simulink model "Model_10_1"  (R2021a)
settings: Solver=VariableStepAuto  StartTime=0.0  StopTime=10  RelTol=1e-3
InitFcn:
  | bx=25; %25
  | bl=50; %50
  | bc=0.1; %0.08
  | 
  | ml=2; %2
  | 
  | mc=0.5;
  | M2=0.5;
  | 
  | mt=5;
  | g=9.81;
  | l_ref=0.3; %0.3
  | l_ini=1;   %1
  | l=l_ini;
  | x_ref=1; %3
  | n1=1; %5
  | n2=1;
  | 
  | L_2=0;  %chieu dai day nang ha
  | 
  | theta1_ini=0*pi/180;
  | theta2_ini=0*pi/180;  %2*pi/180
  | 
  | L_tai=0.1;
  | %ADRC' s parameter caculation
  | %b0 = (1)/(mc+mt+ml);
  | b0=(ml+mc)/(mt*mc+2*ml*mc+mt*ml+ml^2+mc^2); %Enhanced-coupling
  | %k_ESO = 100;
  | k_ESO = 100;
  | T_set  = 3; %5;
  | 
  | s_cl = -5.85/T_set;
  | Kp   = s_cl^2;
  | Kd   = -2*s_cl;
  | 
  | s_ESO = k_ESO*s_cl;
  | l1        = -3*s_ESO;
  | l2        = 3*( s_ESO)^2;
  | l3        = -(s_ESO)^3;
  | 
  | %b1 = (mt+mc)/(mc*ml +mc*mt+ml*mt);
  | b1=1/(ml+mc);
  | k_ESO1 =100; %100
  | T_set1  = 3;   %3
  | s_cl1 = -5.85/T_set1;
  | Kp1   = s_cl1^2;
  | Kd1   = -2*s_cl1;
  | 
  | s_ESO1 = k_ESO1*s_cl1;
  | l11        = -3*s_ESO1;
  | l21        = 3*( s_ESO1)^2;
  | l31        = -(s_ESO1)^3;
  | 
  | 
  | %L1=l_ini;
  | L11=0.65;
  | L2=L_tai;
  | m1=2;
  | %m2=M2;
  | m=5;
  | %Bo input shaping
  | alpha = (1/L11 + 1/L2)*(m1+M2)/m1;
  | beta = (((m1+M2)/m1)^2)*((1/L11 + 1/L2)^2) - 4*(m1+M2)/(m1*L11*L2);
  | w1 = sqrt(g*(alpha - sqrt(beta))/2);
  | w2 = sqrt(g*(alpha + sqrt(beta))/2);
  | damping_ratio = 0;
  | wd1 = w1*sqrt(1-damping_ratio^2);
  | wd2 = w2*sqrt(1-damping_ratio^2);
  | 
  | %wd1=1.998421;
  | %wd2=4.099849;
  | 
  | k = exp(damping_ratio*pi/sqrt(1-damping_ratio^2));
  | 
  | %ETM4_1
  | m_etm4_1 = 0.1;
  | I_etm4_1 = (1+m_etm4_1)*k*k/(k^2 + (1+m_etm4_1)*(k^(4/3)+k^(2/3)) + m_etm4_1);
  | A1_etm4_1 = I_etm4_1/(1+m_etm4_1);
  | A2_etm4_1 = I_etm4_1/(k^(2/3));
  | A3_etm4_1 = I_etm4_1/(k^(4/3));
  | A4_etm4_1 = m_etm4_1*I_etm4_1/((1+m_etm4_1)*(k^2));
  | t1_etm4_1 = (2*pi/3)/wd1;
  | t2_etm4_1 = (4*pi/3)/wd1;
  | t3_etm4_1 = 2*pi/wd1;
  | 
  | %ETM4_2
  | m_etm4_2 = 0.1;
  | I_etm4_2 = (1+m_etm4_2)*k*k/(k^2 + (1+m_etm4_2)*(k^(4/3)+k^(2/3)) + m_etm4_2);
  | A1_etm4_2 = I_etm4_2/(1+m_etm4_2);
  | A2_etm4_2 = I_etm4_2/(k^(2/3));
  | A3_etm4_2 = I_etm4_2/(k^(4/3));
  | A4_etm4_2 = m_etm4_2*I_etm4_2/((1+m_etm4_2)*(k^2));
  | t1_etm4_2 = (2*pi/3)/wd2;
  | t2_etm4_2 = (4*pi/3)/wd2;
  | t3_etm4_2 = 2*pi/wd2;
libraries: neural x1372, simulink x44, simulink_extras x6
(part 1 of 58)
settings Model: Creator=Dao Hieu  LastModifiedBy=Admin

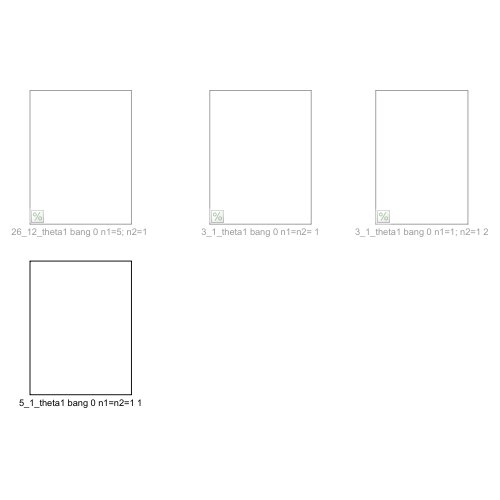
[thumbnail: Simulink's stored preview of the top-level diagram]
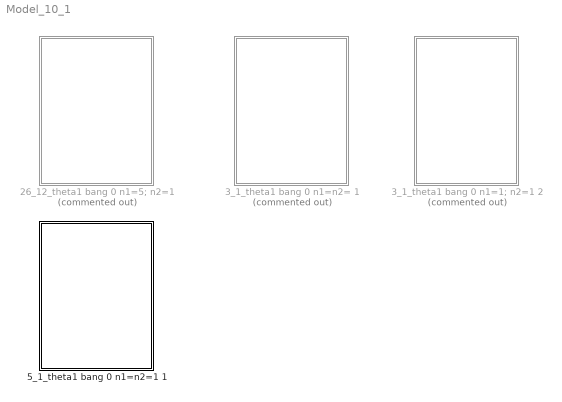
== system Model_10_1 ==
  "26_12_theta1 bang 0 n1=5; n2=1 " : Subsystem  Commented=on
  3_1_theta1 bang 0 n1=1; n2=1 2 : Subsystem  Commented=on
  3_1_theta1 bang 0 n1=n2= 1 : Subsystem  Commented=on
  5_1_theta1 bang 0 n1=n2=1 1 : Subsystem

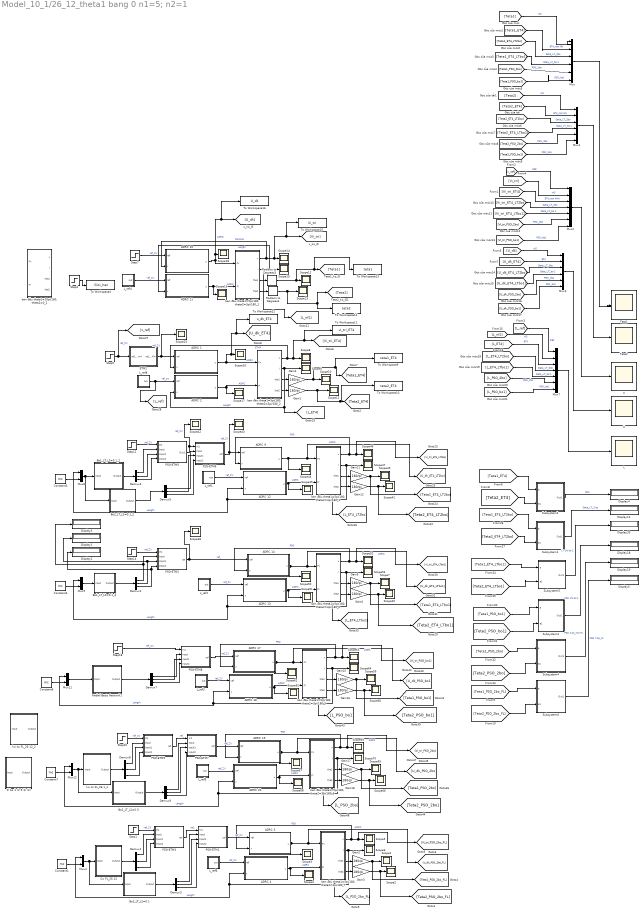
== system Model_10_1/26_12_theta1 bang 0 n1=5; n2=1  ==
  " ban đầu theta1=10pi/180, theta2=0_1" : Subsystem
  ADRC 1 : Subsystem
  ADRC 10 : Subsystem
  ADRC 11 : Subsystem
  ADRC 12 : Subsystem
  ADRC 13 : Subsystem
  ADRC 14 : Subsystem
  ADRC 17 : Subsystem
  ADRC 18 : Subsystem
  ADRC 19 : Subsystem
  ADRC 2 : Subsystem
  ADRC 20 : Subsystem
  ADRC 3 : Subsystem
  ADRC 4 : Subsystem
  ADRC 9 : Subsystem
  Bo1_LT_L2=0.1_2 : Subsystem
      mask help: Radial Basis Network
      mask Display: e = 0.06;c1 = [120 150 230]/255;c2 = ([120 150 230]+0)/383;c3 = ([120 150 230]+128)/383;patch([0 1 1 0],[0 0 1 1],c1);patch([0 1 1 1-e 1-e 0+e],[0 0 1 1-e 0+e 0+e],c2);patch([0 0 1 1-e 0+e 0+e],[0 1 1 1-e 1-e 0+e],c3);plot([0 1 1 0 0],[0 0 1 1 0]);fprintf('NNET');port_label('input',1,' Input');port_label('output',1,'Output ');
  Bo1_LT_L2=0.1_3 : Subsystem
      mask help: Radial Basis Network
      mask Display: e = 0.06;c1 = [120 150 230]/255;c2 = ([120 150 230]+0)/383;c3 = ([120 150 230]+128)/383;patch([0 1 1 0],[0 0 1 1],c1);patch([0 1 1 1-e 1-e 0+e],[0 0 1 1-e 0+e 0+e],c2);patch([0 0 1 1-e 0+e 0+e],[0 1 1 1-e 1-e 0+e],c3);plot([0 1 1 0 0],[0 0 1 1 0]);fprintf('NNET');port_label('input',1,' Input');port_label('output',1,'Output ');
  Bo2_LT_L2=0.1 : Subsystem
      mask help: Radial Basis Network
      mask Display: e = 0.06;c1 = [120 150 230]/255;c2 = ([120 150 230]+0)/383;c3 = ([120 150 230]+128)/383;patch([0 1 1 0],[0 0 1 1],c1);patch([0 1 1 1-e 1-e 0+e],[0 0 1 1-e 0+e 0+e],c2);patch([0 0 1 1-e 0+e 0+e],[0 1 1 1-e 1-e 0+e],c3);plot([0 1 1 0 0],[0 0 1 1 0]);fprintf('NNET');port_label('input',1,' Input');port_label('output',1,'Output ');
  Bo2_LT_L2=0.1_2 : Subsystem
      mask help: Radial Basis Network
      mask Display: e = 0.06;c1 = [120 150 230]/255;c2 = ([120 150 230]+0)/383;c3 = ([120 150 230]+128)/383;patch([0 1 1 0],[0 0 1 1],c1);patch([0 1 1 1-e 1-e 0+e],[0 0 1 1-e 0+e 0+e],c2);patch([0 0 1 1-e 0+e 0+e],[0 1 1 1-e 1-e 0+e],c3);plot([0 1 1 0 0],[0 0 1 1 0]);fprintf('NNET');port_label('input',1,' Input');port_label('output',1,'Output ');
  Bo2_LT_L2=0.3 : Subsystem
      mask help: Radial Basis Network
      mask Display: e = 0.06;c1 = [120 150 230]/255;c2 = ([120 150 230]+0)/383;c3 = ([120 150 230]+128)/383;patch([0 1 1 0],[0 0 1 1],c1);patch([0 1 1 1-e 1-e 0+e],[0 0 1 1-e 0+e 0+e],c2);patch([0 0 1 1-e 0+e 0+e],[0 1 1 1-e 1-e 0+e],c3);plot([0 1 1 0 0],[0 0 1 1 0]);fprintf('NNET');port_label('input',1,' Input');port_label('output',1,'Output ');
  Co FL_25.12 : Subsystem
      mask help: Radial Basis Network
      mask Display: e = 0.06;c1 = [120 150 230]/255;c2 = ([120 150 230]+0)/383;c3 = ([120 150 230]+128)/383;patch([0 1 1 0],[0 0 1 1],c1);patch([0 1 1 1-e 1-e 0+e],[0 0 1 1-e 0+e 0+e],c2);patch([0 0 1 1-e 0+e 0+e],[0 1 1 1-e 1-e 0+e],c3);plot([0 1 1 0 0],[0 0 1 1 0]);fprintf('NNET');port_label('input',1,' Input');port_label('output',1,'Output ');
  Constant{1,3..4,6..7} (5 alike) : Constant  Value=mc
  Demux{1..5,7..9} (8 alike) : Demux  Outputs=3
  Display{1..5,12,18..20} (9 alike) : Display
  ETM2 : Subsystem
  Fl bo 1 (2 5 3) (2) : Subsystem
      mask help: Radial Basis Network
      mask Display: e = 0.06;c1 = [120 150 230]/255;c2 = ([120 150 230]+0)/383;c3 = ([120 150 230]+128)/383;patch([0 1 1 0],[0 0 1 1],c1);patch([0 1 1 1-e 1-e 0+e],[0 0 1 1-e 0+e 0+e],c2);patch([0 0 1 1-e 0+e 0+e],[0 1 1 1-e 1-e 0+e],c3);plot([0 1 1 0 0],[0 0 1 1 0]);fprintf('NNET');port_label('input',1,' Input');port_label('output',1,'Output ');
  Gain{1..6,11..12,15..18} (12 alike) : Gain  Gain=180/pi
  L : Scope
  L_ref1 : Subsystem
  L_ref2 : Subsystem
  L_ref3 : Subsystem
  L_ref4 : Subsystem
  L_ref5 : Subsystem
  L_ref6 : Subsystem
  L_ref8 : Subsystem
  Mux : Mux  Inputs=6
  Mux1 : Mux  Inputs=6
  Mux{4,8..9,11..12} (5 alike) : Mux  Inputs=2
  Mux2 : Mux  Inputs=7
  Mux3 : Mux  Inputs=6
  Mux7 : Mux  Inputs=7
  PSO-ETM1 : Subsystem
  PSO-ETM2 : Subsystem
  PSO-ETM3 : Subsystem
  PSO-ETM5 : Subsystem
  PSO-ETM6 : Subsystem
  PSO-ETM7 : Subsystem
  PSO-ETM8 : Subsystem
  PSO-ETM9 : Subsystem
  Radial Basis Network1 : Subsystem
      mask help: Radial Basis Network
      mask Display: e = 0.06;c1 = [120 150 230]/255;c2 = ([120 150 230]+0)/383;c3 = ([120 150 230]+128)/383;patch([0 1 1 0],[0 0 1 1],c1);patch([0 1 1 1-e 1-e 0+e],[0 0 1 1-e 0+e 0+e],c2);patch([0 0 1 1-e 0+e 0+e],[0 1 1 1-e 1-e 0+e],c3);plot([0 1 1 0 0],[0 0 1 1 0]);fprintf('NNET');port_label('input',1,' Input');port_label('output',1,'Output ');
  Radians to Degrees3 : simulink_extras/Transformations/Radians to Degrees
  Radians to Degrees4 : simulink_extras/Transformations/Radians to Degrees
  Scope{1..20,23,40..48,50..53,59..70} (46 alike) : Scope
  Step{1,5,7,12,14,18,20} (7 alike) : Step  Time=0  After=x_ref  SampleTime=0
  Step3 : Step  Time=0  After=10  SampleTime=0
  Subsystem1 : Subsystem
  Subsystem2 : Subsystem
  Subsystem3 : Subsystem
  Subsystem4 : Subsystem
  Subsystem5 : Subsystem
  Subsystem6 : Subsystem
  Teta1 : Scope
  Teta2 : Scope
  To Workspace10 : ToWorkspace  VariableName=teta2_ET4  SaveFormat=Timeseries  SampleTime=-1
  To Workspace11 : ToWorkspace  VariableName=vi_tri_ET4  SaveFormat=Timeseries  SampleTime=-1
  To Workspace12 : ToWorkspace  VariableName=u_dk_ET4  SaveFormat=Timeseries  SampleTime=-1
  To Workspace13 : ToWorkspace  VariableName=teta1  SaveFormat=Timeseries  SampleTime=-1
  To Workspace14 : ToWorkspace  VariableName=teta2  SaveFormat=Timeseries  SampleTime=-1
  To Workspace15 : ToWorkspace  VariableName=Vi_tri  SaveFormat=Timeseries  SampleTime=-1
  To Workspace16 : ToWorkspace  VariableName=U_dk  SaveFormat=Timeseries  SampleTime=-1
  To Workspace4 : ToWorkspace  VariableName=Gioi_han  SaveFormat=Timeseries  SampleTime=-1
  To Workspace9 : ToWorkspace  VariableName=teta1_ET4  SaveFormat=Timeseries  SampleTime=-1
  U : Scope
  X : Scope
  "ban đầu theta1=5pi/180, theta2=3pi/180_1" : Subsystem
  "ban đầu theta1=5pi/180, theta2=3pi/180_2" : Subsystem
  "ban đầu theta1=5pi/180, theta2=3pi/180_3" : Subsystem
  "ban đầu theta1=5pi/180, theta2=3pi/180_4" : Subsystem
  "ban đầu theta1=5pi/180, theta2=3pi/180_5" : Subsystem
  "ban đầu theta1=5pi/180, theta2=3pi/180_6" : Subsystem
  "ban đầu theta1=5pi/180, theta2=3pi/180_7" : Subsystem
  ko co FL_25.12_2 : Subsystem
      mask help: Radial Basis Network
      mask Display: e = 0.06;c1 = [120 150 230]/255;c2 = ([120 150 230]+0)/383;c3 = ([120 150 230]+128)/383;patch([0 1 1 0],[0 0 1 1],c1);patch([0 1 1 1-e 1-e 0+e],[0 0 1 1-e 0+e 0+e],c2);patch([0 0 1 1-e 0+e 0+e],[0 1 1 1-e 1-e 0+e],c3);plot([0 1 1 0 0],[0 0 1 1 0]);fprintf('NNET');port_label('input',1,' Input');port_label('output',1,'Output ');
  ko co FL_26.1_1 : Subsystem
      mask help: Radial Basis Network
      mask Display: e = 0.06;c1 = [120 150 230]/255;c2 = ([120 150 230]+0)/383;c3 = ([120 150 230]+128)/383;patch([0 1 1 0],[0 0 1 1],c1);patch([0 1 1 1-e 1-e 0+e],[0 0 1 1-e 0+e 0+e],c2);patch([0 0 1 1-e 0+e 0+e],[0 1 1 1-e 1-e 0+e],c3);plot([0 1 1 0 0],[0 0 1 1 0]);fprintf('NNET');port_label('input',1,' Input');port_label('output',1,'Output ');
  wires:
  ADRC 2/1(u) -> "ban đầu theta1=5pi/180, theta2=3pi/180_2"/2(Fl), Scope17/1  "ADRC"
  ADRC 11/1(u) -> "ban đầu theta1=5pi/180, theta2=3pi/180_1"/2(Fl), Scope19/1  "ADRC"
  ADRC 1/1(u) -> "ban đầu theta1=5pi/180, theta2=3pi/180_2"/1(Fx), To Workspace12/1, [U_dk_ET4], Scope16/1  "ADRC"
  "ban đầu theta1=5pi/180, theta2=3pi/180_2"/1(x) -> ADRC 1/2(x), To Workspace11/1, [Vi_tri_ET4], Scope8/1  "ETM4"
  "ban đầu theta1=5pi/180, theta2=3pi/180_1"/3(the1) -> Radians to Degrees3/1
  "ban đầu theta1=5pi/180, theta2=3pi/180_2"/2(l) -> [L_ET4], ADRC 2/2(x), Scope9/1  "Length"
  "ban đầu theta1=5pi/180, theta2=3pi/180_1"/1(x) -> ADRC 10/2(x), To Workspace15/1, [Vi_tri], Scope14/1  "Position"
  L_ref4/1(out) -> ADRC 11/1(ref)  "ref_ZV"
  L_ref8/1(out) -> [L_ref], ADRC 2/1(ref)  "ref_ZV"
  "ban đầu theta1=5pi/180, theta2=3pi/180_1"/2(l) -> Scope15/1, ADRC 11/2(x), [L_nIS]  "Length"
  Step7/1 -> ADRC 10/1(ref)  "ref_ZV"
  Gain4/1 -> To Workspace9/1, [Teta1_ET4], Scope10/1
  ETM2/1(ref_ETM4) -> ADRC 1/1(ref), Scope23/1  "ref_ZV"
  Step5/1 -> [x_ref], ETM2/1(ref_ETm4)  "ref_ZV"
  ADRC 10/1(u) -> "ban đầu theta1=5pi/180, theta2=3pi/180_1"/1(Fx), To Workspace16/1, [U_dk], Scope18/1  "ADRC"
  Radians to Degrees3/1 -> To Workspace13/1, [Teta1], Scope12/1
  "ban đầu theta1=5pi/180, theta2=3pi/180_1"/4(the2) -> Radians to Degrees4/1
  "ban đầu theta1=5pi/180, theta2=3pi/180_2"/3(the1) -> Gain4/1
  Gain1/1 -> To Workspace10/1, [Teta2_ET4], Scope11/1
  "ban đầu theta1=5pi/180, theta2=3pi/180_2"/4(the2) -> Gain1/1
  Radians to Degrees4/1 -> [Teta2], To Workspace14/1, Scope13/1
  [Teta2] -> Mux1/1  "nIS"
  [U_dk] -> Mux3/1  "nIS"
  [U_dk_ET4] -> Mux3/2  "ET4"
  [Teta2_ET4] -> Mux1/2  "ET4_non NN"
  [Teta1] -> Mux/1  "nIS"
  Mux2/1 -> X/1
  Mux/1 -> Teta1/1
  Mux1/1 -> Teta2/1
  Mux3/1 -> U/1
  [Teta1_ET4] -> Mux/2  "ET4_non NN"
  Step3/1 -> To Workspace4/1
  Mux7/1 -> L/1
  "ban đầu theta1=5pi/180, theta2=3pi/180_3"/3(the1) -> Gain11/1
  "ban đầu theta1=5pi/180, theta2=3pi/180_3"/1(x) -> ADRC 9/2(x), [Vi_tri_ET4_LT2bo], Scope46/1  "PSO"
  ADRC 9/1(u) -> "ban đầu theta1=5pi/180, theta2=3pi/180_3"/1(Fx), [U_dk_ET4_LT2bo], Scope44/1  "ADRC"
  Gain12/1 -> [Teta2_ET4_LT2bo], Scope41/1
  ADRC 12/1(u) -> "ban đầu theta1=5pi/180, theta2=3pi/180_3"/2(Fl), Scope45/1  "ADRC"
  Demux4/3 -> PSO-ETM5/4(Input2)
  PSO-ETM6/1(ref) -> ADRC 9/1(ref), Scope43/1  "ref_ZV"
  "ban đầu theta1=5pi/180, theta2=3pi/180_3"/4(the2) -> Gain12/1
  Step12/1 -> PSO-ETM5/1(In1)  "ref_ZV"
  Demux5/2 -> PSO-ETM6/3(Input1)
  Demux4/2 -> PSO-ETM5/3(Input1)
  Constant3/1 -> Mux8/2
  Gain11/1 -> [Teta1_ET4_LT2bo], Scope40/1
  Demux5/3 -> PSO-ETM6/4(Input2)
  "ban đầu theta1=5pi/180, theta2=3pi/180_3"/2(l) -> Scope47/1, [L_ET4_LT2bo], ADRC 12/2(x), Mux8/1  "Length"
  Bo2_LT_L2=0.1_2/1(Output) -> Demux5/1
  PSO-ETM5/1(Out1) -> PSO-ETM6/1(In1), Scope42/1  "ref_ZV"
  Demux4/1 -> PSO-ETM5/2(Input)
  Mux8/1 -> Bo2_LT_L2=0.1_2/1(Input), Bo1_LT_L2=0.1_2/1(Input)
  Demux5/1 -> PSO-ETM6/2(Input)
  L_ref1/1(out) -> ADRC 12/1(ref)  "ref_ZV"
  Demux2/1 -> Display3/1, PSO-ETM2/2(Input)
  ADRC 13/1(u) -> "ban đầu theta1=5pi/180, theta2=3pi/180_4"/2(Fl), Scope51/1  "ADRC"
  Constant4/1 -> Mux9/2
  "ban đầu theta1=5pi/180, theta2=3pi/180_4"/2(l) -> Scope53/1, [L_ET4_LTbo1], ADRC 13/2(x), Mux9/1  "Length"
  Demux2/2 -> Display1/1, PSO-ETM2/3(Input1)
  L_ref2/1(out) -> ADRC 13/1(ref)  "ref_ZV"
  Step14/1 -> PSO-ETM2/1(In1)  "ref_ZV"
  Mux9/1 -> Bo1_LT_L2=0.1_3/1(Input)
  Demux2/3 -> Display2/1, PSO-ETM2/4(Input2)
  "ban đầu theta1=5pi/180, theta2=3pi/180_4"/4(the2) -> Gain6/1
  PSO-ETM2/1(ref) -> ADRC 14/1(ref), Scope48/1  "ref_"
  Gain5/1 -> [Teta1_ET4_LTbo1], Scope7/1
  Gain6/1 -> [Teta2_ET4_LTbo1], Scope20/1
  "ban đầu theta1=5pi/180, theta2=3pi/180_4"/3(the1) -> Gain5/1
  ADRC 14/1(u) -> Scope50/1, "ban đầu theta1=5pi/180, theta2=3pi/180_4"/1(Fx), [U_dk_ET4_LTbo1]  "ADRC"
  "ban đầu theta1=5pi/180, theta2=3pi/180_4"/1(x) -> ADRC 14/2(x), [Vi_tri_ET4_LTbo1], Scope52/1  "PSO"
  Bo1_LT_L2=0.1_3/1(Output) -> Demux2/1
  Demux7/3 -> PSO-ETM8/4(Input2)
  Demux7/1 -> PSO-ETM8/2(Input)
  Gain16/1 -> [Teta2_PSO_bo1], Scope60/1
  "ban đầu theta1=5pi/180, theta2=3pi/180_5"/4(the2) -> Gain16/1
  "ban đầu theta1=5pi/180, theta2=3pi/180_5"/3(the1) -> Gain15/1
  Constant6/1 -> Mux11/2
  Gain15/1 -> [Teta1_PSO_bo1], Scope59/1
  Demux7/2 -> PSO-ETM8/3(Input1)
  "ban đầu theta1=5pi/180, theta2=3pi/180_5"/2(l) -> Scope64/1, [L_PSO_bo1], ADRC 18/2(x), Mux11/1  "Length"
  L_ref3/1(out) -> ADRC 18/1(ref)  "ref_ZV"
  PSO-ETM8/1(ref) -> ADRC 17/1(ref)  "ref_ZV"
  Step18/1 -> PSO-ETM8/1(In1)  "ref_ZV"
  ADRC 17/1(u) -> Scope61/1, "ban đầu theta1=5pi/180, theta2=3pi/180_5"/1(Fx), [U_dk_PSO_bo1]  "ADRC"
  "ban đầu theta1=5pi/180, theta2=3pi/180_5"/1(x) -> ADRC 17/2(x), [Vi_tri_PSO_bo1], Scope63/1  "PSO"
  ADRC 18/1(u) -> "ban đầu theta1=5pi/180, theta2=3pi/180_5"/2(Fl), Scope62/1  "ADRC"
  "ban đầu theta1=5pi/180, theta2=3pi/180_6"/1(x) -> ADRC 19/2(x), [Vi_tri_PSO_2bo], Scope69/1  "PSO"
  ADRC 19/1(u) -> Scope67/1, "ban đầu theta1=5pi/180, theta2=3pi/180_6"/1(Fx), [U_dk_PSO_2bo]  "ADRC"
  "ban đầu theta1=5pi/180, theta2=3pi/180_6"/2(l) -> Scope70/1, [L_PSO_2bo], ADRC 20/2(x), Mux12/1  "Length"
  L_ref5/1(out) -> ADRC 20/1(ref)  "ref_ZV"
  Step20/1 -> PSO-ETM9/1(In1)  "ref_ZV"
  "ban đầu theta1=5pi/180, theta2=3pi/180_6"/4(the2) -> Gain18/1
  "ban đầu theta1=5pi/180, theta2=3pi/180_6"/3(the1) -> Gain17/1
  Gain17/1 -> [Teta1_PSO_2bo], Scope65/1
  Gain18/1 -> [Teta2_PSO_2bo], Scope66/1
  Constant7/1 -> Mux12/2
  ADRC 20/1(u) -> "ban đầu theta1=5pi/180, theta2=3pi/180_6"/2(Fl), Scope68/1  "ADRC"
  Bo1_LT_L2=0.1_2/1(Output) -> Demux4/1
  Radial Basis Network1/1(Output) -> Demux7/1
  Mux11/1 -> Radial Basis Network1/1(Input)
  Demux8/1 -> PSO-ETM9/2(Input)
  Demux8/2 -> PSO-ETM9/3(Input1)
  Demux8/3 -> PSO-ETM9/4(Input2)
  [Teta1_ET4_LTbo1] -> Subsystem5/1(e)
  Subsystem4/1(Out1) -> Display19/1  "PSO 2 bo_non FL"
  [Teta2_ET4_LT2bo] -> Subsystem1/2(e1)
  [Teta2_PSO_bo1] -> Subsystem3/2(e1)
  Subsystem5/1(Out1) -> Display20/1  "LT chi bo 1"
  [Teta2_ET4_LTbo1] -> Subsystem5/2(e1)
  [Teta1_PSO_2bo] -> Subsystem4/1(e)
  [Teta2_PSO_2bo] -> Subsystem4/2(e1)
  Subsystem1/1(Out1) -> Display12/1  "Data_LT_2 bo"
  Subsystem3/1(Out1) -> Display18/1  "PSO chi bo 1"
  [Teta1_PSO_bo1] -> Subsystem3/1(e)
  [Teta1_ET4_LT2bo] -> Subsystem1/1(e)
  Bo2_LT_L2=0.3/1(Output) -> Demux9/1
  Demux9/2 -> PSO-ETM7/3(Input1)
  Mux12/1 -> ko co FL_26.1_1/1(Input), Bo2_LT_L2=0.3/1(Input)
  Demux9/3 -> PSO-ETM7/4(Input2)
  Demux9/1 -> PSO-ETM7/2(Input)
  PSO-ETM9/1(ref) -> PSO-ETM7/1(In1)  "ref_"
  PSO-ETM7/1(ref) -> ADRC 19/1(ref)  "ref_ZV"
  [Teta1_ET4_LT2bo] -> Mux/3  "Data_LT_2bo"
  [Teta1_ET4_LTbo1] -> Mux/4  "Data_LT_bo 1"
  [Teta1_PSO_2bo] -> Mux/5  "PSO_2bo"
  [Teta1_PSO_bo1] -> Mux/6  "PSO_bo1"
  [Teta2_ET4_LT2bo] -> Mux1/3  "Data_LT_2bo"
  [Teta2_ET4_LTbo1] -> Mux1/4  "Data_LT_bo 1"
  [Teta2_PSO_2bo] -> Mux1/5  "PSO_2bo"
  [Teta2_PSO_bo1] -> Mux1/6  "PSO_bo1"
  [x_ref] -> Mux2/1  "REF"
  [Vi_tri] -> Mux2/2  "nIS"
  [Vi_tri_ET4] -> Mux2/3  "ET4_non ANN"
  [Vi_tri_ET4_LT2bo] -> Mux2/4  "Data_LT_2bo"
  [Vi_tri_ET4_LTbo1] -> Mux2/5  "Data_LT_bo 1"
  [Vi_tri_PSO_2bo] -> Mux2/6  "PSO_2bo"
  [Vi_tri_PSO_bo1] -> Mux2/7  "PSO_bo1"
  [U_dk_ET4_LT2bo] -> Mux3/3  "Data_LT_2bo"
  [U_dk_ET4_LTbo1] -> Mux3/4  "Data_LT_bo 1"
  [U_dk_PSO_2bo] -> Mux3/5  "PSO_2bo"
  [U_dk_PSO_bo1] -> Mux3/6  "PSO_bo1"
  [L_ref] -> Mux7/1  "REF"
  [L_nIS] -> Mux7/2  "nIS"
  [L_ET4] -> Mux7/3  "ET4"
  [L_ET4_LT2bo] -> Mux7/4  "Data_LT_2bo"
  [L_ET4_LTbo1] -> Mux7/5  "Data_LT_bo 1"
  [L_PSO_2bo] -> Mux7/6  "PSO_2bo"
  [L_PSO_bo1] -> Mux7/7  "PSO_bo1"
  [Teta1_ET4] -> Subsystem2/1(e)
  [Teta2_ET4] -> Subsystem2/2(e1)
  Subsystem2/1(Out1) -> Display4/1  "ET4"
  ko co FL_26.1_1/1(Output) -> Demux8/1
  "ban đầu theta1=5pi/180, theta2=3pi/180_7"/4(the2) -> Gain3/1
  Demux1/2 -> PSO-ETM3/3(Input1)
  PSO-ETM3/1(ref) -> PSO-ETM1/1(In1)  "ref_"
  ADRC 4/1(u) -> "ban đầu theta1=5pi/180, theta2=3pi/180_7"/2(Fl), Scope4/1  "ADRC"
  Constant1/1 -> Mux4/2
  Co FL_25.12/1(Output) -> Demux1/1
  Demux1/1 -> PSO-ETM3/2(Input)
  Demux1/3 -> PSO-ETM3/4(Input2)
  Gain3/1 -> [Teta2_PSO_2bo_FL], Scope2/1
  L_ref6/1(out) -> ADRC 4/1(ref)  "ref_ZV"
  Gain2/1 -> [Teta1_PSO_2bo_FL], Scope1/1
  "ban đầu theta1=5pi/180, theta2=3pi/180_7"/2(l) -> Scope6/1, [L_PSO_2bo_FL], ADRC 4/2(x), Mux4/1  "Length"
  "ban đầu theta1=5pi/180, theta2=3pi/180_7"/3(the1) -> Gain2/1
  "ban đầu theta1=5pi/180, theta2=3pi/180_7"/1(x) -> ADRC 3/2(x), [Vi_tri_PSO_2bo_FL], Scope5/1  "PSO"
  Step1/1 -> PSO-ETM3/1(In1)  "ref_ZV"
  Demux3/1 -> PSO-ETM1/2(Input)
  PSO-ETM1/1(ref) -> ADRC 3/1(ref)  "ref_ZV"
  ADRC 3/1(u) -> Scope3/1, "ban đầu theta1=5pi/180, theta2=3pi/180_7"/1(Fx), [U_dk_PSO_2bo_FL]  "ADRC"
  Demux3/3 -> PSO-ETM1/4(Input2)
  Mux4/1 -> Co FL_25.12/1(Input), Bo2_LT_L2=0.1/1(Input)
  Demux3/2 -> PSO-ETM1/3(Input1)
  Bo2_LT_L2=0.1/1(Output) -> Demux3/1
  [Teta2_PSO_2bo_FL] -> Subsystem6/2(e1)
  Subsystem6/1(Out1) -> Display5/1  "PSO 2 bo_FL"
  [Teta1_PSO_2bo_FL] -> Subsystem6/1(e)

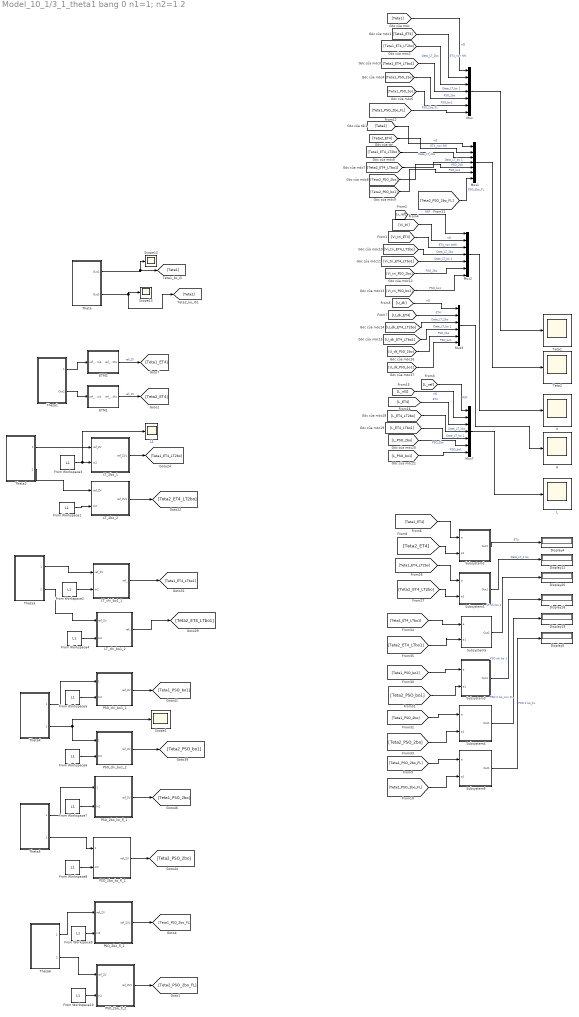
== system Model_10_1/3_1_theta1 bang 0 n1=1; n2=1 2 ==
  Display{4..5,12,18..20} (6 alike) : Display
  ETM1 : Subsystem
  ETM2 : Subsystem
  From Workspace{1..10} (10 alike) : FromWorkspace  VariableName=L1  SampleTime=5e-3
  L : Scope
  L1 : Scope
  LT_2bo_1 : Subsystem
  LT_2bo_2 : Subsystem
  LT_chi_bo1_1 : Subsystem
  LT_chi_bo1_2 : Subsystem
  Mux{,1..2,7} (4 alike) : Mux  Inputs=7
  Mux3 : Mux  Inputs=6
  PSO_2bo_fl_1 : Subsystem
  PSO_2bo_fl_2 : Subsystem
  PSO_2bo_ko_fl_1 : Subsystem
  PSO_2bo_ko_fl_2 : Subsystem
  PSO_chi_bo1_1 : Subsystem
  PSO_chi_bo1_2 : Subsystem
  Scope1 : Scope
  Scope12 : Scope
  Scope13 : Scope
  Subsystem1 : Subsystem
  Subsystem2 : Subsystem
  Subsystem3 : Subsystem
  Subsystem4 : Subsystem
  Subsystem5 : Subsystem
  Subsystem6 : Subsystem
  Teta1 : Scope
  Teta2 : Scope
  Theta : Subsystem
  Theta1 : Subsystem
  Theta2 : Subsystem
  Theta3 : Subsystem
  Theta4 : Subsystem
  Theta5 : Subsystem
  Theta6 : Subsystem
  U : Scope
  X : Scope
  wires:
  [Teta2] -> Mux1/1  "nIS"
  [U_dk] -> Mux3/1  "nIS"
  [U_dk_ET4] -> Mux3/2  "ET4"
  [Teta2_ET4] -> Mux1/2  "ET4_non NN"
  [Teta1] -> Mux/1  "nIS"
  Mux2/1 -> X/1
  Mux/1 -> Teta1/1
  Mux1/1 -> Teta2/1
  Mux3/1 -> U/1
  [Teta1_ET4] -> Mux/2  "ET4_non NN"
  Mux7/1 -> L/1
  [Teta1_ET4_LTbo1] -> Subsystem5/1(e)
  Subsystem4/1(Out1) -> Display19/1  "PSO 2 bo_non FL"
  [Teta2_ET4_LT2bo] -> Subsystem1/2(e1)
  [Teta2_PSO_bo1] -> Subsystem3/2(e1)
  Subsystem5/1(Out1) -> Display20/1  "LT chi bo 1"
  [Teta2_ET4_LTbo1] -> Subsystem5/2(e1)
  [Teta1_PSO_2bo] -> Subsystem4/1(e)
  [Teta2_PSO_2bo] -> Subsystem4/2(e1)
  Subsystem1/1(Out1) -> Display12/1  "Data_LT_2 bo"
  Subsystem3/1(Out1) -> Display18/1  "PSO chi bo 1"
  [Teta1_PSO_bo1] -> Subsystem3/1(e)
  [Teta1_ET4_LT2bo] -> Subsystem1/1(e)
  [Teta1_ET4_LT2bo] -> Mux/3  "Data_LT_2bo"
  [Teta1_ET4_LTbo1] -> Mux/4  "Data_LT_bo 1"
  [Teta1_PSO_2bo] -> Mux/5  "PSO_2bo"
  [Teta1_PSO_bo1] -> Mux/6  "PSO_bo1"
  [Teta2_ET4_LT2bo] -> Mux1/3  "Data_LT_2bo"
  [Teta2_ET4_LTbo1] -> Mux1/4  "Data_LT_bo 1"
  [Teta2_PSO_2bo] -> Mux1/5  "PSO_2bo"
  [Teta2_PSO_bo1] -> Mux1/6  "PSO_bo1"
  [x_ref] -> Mux2/1  "REF"
  [Vi_tri] -> Mux2/2  "nIS"
  [Vi_tri_ET4] -> Mux2/3  "ET4_non ANN"
  [Vi_tri_ET4_LT2bo] -> Mux2/4  "Data_LT_2bo"
  [Vi_tri_ET4_LTbo1] -> Mux2/5  "Data_LT_bo 1"
  [Vi_tri_PSO_2bo] -> Mux2/6  "PSO_2bo"
  [Vi_tri_PSO_bo1] -> Mux2/7  "PSO_bo1"
  [U_dk_ET4_LT2bo] -> Mux3/3  "Data_LT_2bo"
  [U_dk_ET4_LTbo1] -> Mux3/4  "Data_LT_bo 1"
  [U_dk_PSO_2bo] -> Mux3/5  "PSO_2bo"
  [U_dk_PSO_bo1] -> Mux3/6  "PSO_bo1"
  [L_ref] -> Mux7/1  "REF"
  [L_nIS] -> Mux7/2  "nIS"
  [L_ET4] -> Mux7/3  "ET4"
  [L_ET4_LT2bo] -> Mux7/4  "Data_LT_2bo"
  [L_ET4_LTbo1] -> Mux7/5  "Data_LT_bo 1"
  [L_PSO_2bo] -> Mux7/6  "PSO_2bo"
  [L_PSO_bo1] -> Mux7/7  "PSO_bo1"
  [Teta1_ET4] -> Subsystem2/1(e)
  [Teta2_ET4] -> Subsystem2/2(e1)
  Subsystem2/1(Out1) -> Display4/1  "ET4"
  [Teta2_PSO_2bo_FL] -> Subsystem6/2(e1)
  Subsystem6/1(Out1) -> Display5/1  "PSO 2 bo_FL"
  [Teta1_PSO_2bo_FL] -> Subsystem6/1(e)
  [Teta1_PSO_2bo_FL] -> Mux/7  "PSO_2bo_FL"
  [Teta2_PSO_2bo_FL] -> Mux1/7  "PSO_2bo_FL"
  Theta/2(Out2) -> [Teta2], Scope13/1
  Theta/1(Out1) -> Scope12/1, [Teta1]
  Theta1/1(1) -> ETM2/1(ref_ETm4)
  Theta1/2(Out2) -> ETM1/1(ref_ETm4)
  ETM2/1(ref_ETM4) -> [Teta1_ET4]  "ref_ZV"
  ETM1/1(ref_ETM4) -> [Teta2_ET4]  "ref_ZV"
  From Workspace3/1 -> L1/1, LT_2bo_1/2(In2)
  Theta2/1(1) -> LT_2bo_1/1(ref_ZV)
  Theta2/2(2) -> LT_2bo_2/1(ref_ZV)
  From Workspace1/1 -> LT_2bo_2/2(In2)
  LT_2bo_1/1(ref_ZV1) -> [Teta1_ET4_LT2bo]
  LT_2bo_2/1(ref_ZV1) -> [Teta2_ET4_LT2bo]
  Theta3/1(1) -> LT_chi_bo1_1/1(ref_ZV)
  From Workspace2/1 -> LT_chi_bo1_1/2(In2)
  LT_chi_bo1_1/1(ref_) -> [Teta1_ET4_LTbo1]
  From Workspace4/1 -> LT_chi_bo1_2/2(In2)
  Theta3/2(2) -> LT_chi_bo1_2/1(ref_ZV)
  LT_chi_bo1_2/1(ref_) -> [Teta2_ET4_LTbo1]
  From Workspace5/1 -> PSO_chi_bo1_1/2(In2)
  From Workspace6/1 -> PSO_chi_bo1_2/2(In2)
  PSO_chi_bo1_1/1(ref_ZV) -> [Teta1_PSO_bo1]
  PSO_chi_bo1_2/1(ref_ZV) -> [Teta2_PSO_bo1]
  Theta4/1(1) -> PSO_chi_bo1_1/1(1)
  Theta4/2(2) -> PSO_chi_bo1_2/1(1), Scope1/1
  From Workspace7/1 -> PSO_2bo_ko_fl_1/2(In2)
  From Workspace8/1 -> PSO_2bo_ko_fl_2/2(In2)
  Theta5/1(1) -> PSO_2bo_ko_fl_1/1(1)
  Theta5/2(2) -> PSO_2bo_ko_fl_2/1(1)
  PSO_2bo_ko_fl_1/1(ref_ZV) -> [Teta1_PSO_2bo]
  PSO_2bo_ko_fl_2/1(ref_ZV) -> [Teta2_PSO_2bo]
  From Workspace9/1 -> PSO_2bo_fl_1/2(In2)
  From Workspace10/1 -> PSO_2bo_fl_2/2(In2)
  Theta6/1(1) -> PSO_2bo_fl_1/1(ref_ZV)
  Theta6/2(2) -> PSO_2bo_fl_2/1(ref_ZV)
  PSO_2bo_fl_1/1(ref_ZV1) -> [Teta1_PSO_2bo_FL]
  PSO_2bo_fl_2/1(ref_ZV1) -> [Teta2_PSO_2bo_FL]

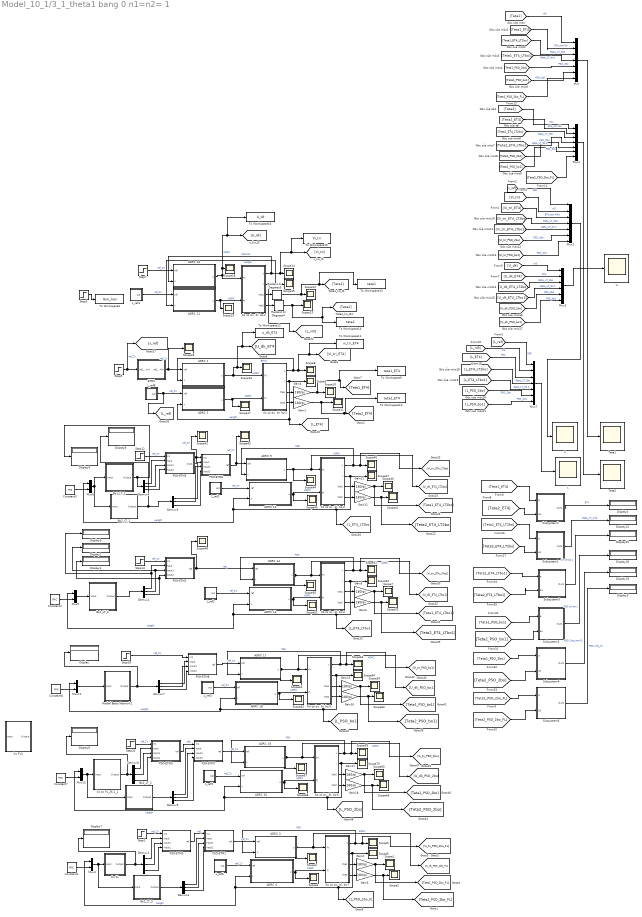
== system Model_10_1/3_1_theta1 bang 0 n1=n2= 1 ==
  ADRC 1 : Subsystem
  ADRC 10 : Subsystem
  ADRC 11 : Subsystem
  ADRC 12 : Subsystem
  ADRC 13 : Subsystem
  ADRC 14 : Subsystem
  ADRC 17 : Subsystem
  ADRC 18 : Subsystem
  ADRC 19 : Subsystem
  ADRC 2 : Subsystem
  ADRC 20 : Subsystem
  ADRC 3 : Subsystem
  ADRC 4 : Subsystem
  ADRC 9 : Subsystem
  Bo1_LT_1 : Subsystem
      mask help: Radial Basis Network
      mask Display: e = 0.06;c1 = [120 150 230]/255;c2 = ([120 150 230]+0)/383;c3 = ([120 150 230]+128)/383;patch([0 1 1 0],[0 0 1 1],c1);patch([0 1 1 1-e 1-e 0+e],[0 0 1 1-e 0+e 0+e],c2);patch([0 0 1 1-e 0+e 0+e],[0 1 1 1-e 1-e 0+e],c3);plot([0 1 1 0 0],[0 0 1 1 0]);fprintf('NNET');port_label('input',1,' Input');port_label('output',1,'Output ');
  Bo1_LT_2 : Subsystem
      mask help: Radial Basis Network
      mask Display: e = 0.06;c1 = [120 150 230]/255;c2 = ([120 150 230]+0)/383;c3 = ([120 150 230]+128)/383;patch([0 1 1 0],[0 0 1 1],c1);patch([0 1 1 1-e 1-e 0+e],[0 0 1 1-e 0+e 0+e],c2);patch([0 0 1 1-e 0+e 0+e],[0 1 1 1-e 1-e 0+e],c3);plot([0 1 1 0 0],[0 0 1 1 0]);fprintf('NNET');port_label('input',1,' Input');port_label('output',1,'Output ');
  Bo2_LT_1 : Subsystem
      mask help: Radial Basis Network
      mask Display: e = 0.06;c1 = [120 150 230]/255;c2 = ([120 150 230]+0)/383;c3 = ([120 150 230]+128)/383;patch([0 1 1 0],[0 0 1 1],c1);patch([0 1 1 1-e 1-e 0+e],[0 0 1 1-e 0+e 0+e],c2);patch([0 0 1 1-e 0+e 0+e],[0 1 1 1-e 1-e 0+e],c3);plot([0 1 1 0 0],[0 0 1 1 0]);fprintf('NNET');port_label('input',1,' Input');port_label('output',1,'Output ');
  Bo2_LT_2 : Subsystem
      mask help: Radial Basis Network
      mask Display: e = 0.06;c1 = [120 150 230]/255;c2 = ([120 150 230]+0)/383;c3 = ([120 150 230]+128)/383;patch([0 1 1 0],[0 0 1 1],c1);patch([0 1 1 1-e 1-e 0+e],[0 0 1 1-e 0+e 0+e],c2);patch([0 0 1 1-e 0+e 0+e],[0 1 1 1-e 1-e 0+e],c3);plot([0 1 1 0 0],[0 0 1 1 0]);fprintf('NNET');port_label('input',1,' Input');port_label('output',1,'Output ');
  Bo2_LT_3 : Subsystem
      mask help: Radial Basis Network
      mask Display: e = 0.06;c1 = [120 150 230]/255;c2 = ([120 150 230]+0)/383;c3 = ([120 150 230]+128)/383;patch([0 1 1 0],[0 0 1 1],c1);patch([0 1 1 1-e 1-e 0+e],[0 0 1 1-e 0+e 0+e],c2);patch([0 0 1 1-e 0+e 0+e],[0 1 1 1-e 1-e 0+e],c3);plot([0 1 1 0 0],[0 0 1 1 0]);fprintf('NNET');port_label('input',1,' Input');port_label('output',1,'Output ');
  Co FL : Subsystem
      mask help: Radial Basis Network
      mask Display: e = 0.06;c1 = [120 150 230]/255;c2 = ([120 150 230]+0)/383;c3 = ([120 150 230]+128)/383;patch([0 1 1 0],[0 0 1 1],c1);patch([0 1 1 1-e 1-e 0+e],[0 0 1 1-e 0+e 0+e],c2);patch([0 0 1 1-e 0+e 0+e],[0 1 1 1-e 1-e 0+e],c3);plot([0 1 1 0 0],[0 0 1 1 0]);fprintf('NNET');port_label('input',1,' Input');port_label('output',1,'Output ');
  Constant{1,3..4,6..7} (5 alike) : Constant  Value=mc
  Demux{1..5,7..9} (8 alike) : Demux  Outputs=3
  Display{,1..9,12,18..20} (14 alike) : Display
  ETM2 : Subsystem
  Gain{1..6,11..12,15..18} (12 alike) : Gain  Gain=180/pi
  "Ko co bx, bl, bc-1" : Subsystem
  "Ko co bx, bl, bc-2" : Subsystem
  "Ko co bx, bl, bc-3" : Subsystem
  "Ko co bx, bl, bc-4" : Subsystem
  "Ko co bx, bl, bc-5" : Subsystem
  "Ko co bx, bl, bc-6" : Subsystem
  "Ko co bx, bl, bc-7" : Subsystem
  L : Scope
  L_ref1 : Subsystem
  L_ref2 : Subsystem
  L_ref3 : Subsystem
  L_ref4 : Subsystem
  L_ref5 : Subsystem
  L_ref6 : Subsystem
  L_ref8 : Subsystem
  Mux{,1..2,7} (4 alike) : Mux  Inputs=7
  Mux{4,8..9,11..12} (5 alike) : Mux  Inputs=2
  Mux3 : Mux  Inputs=6
  PSO-ETM1 : Subsystem
  PSO-ETM2 : Subsystem
  PSO-ETM3 : Subsystem
  PSO-ETM5 : Subsystem
  PSO-ETM6 : Subsystem
  PSO-ETM7 : Subsystem
  PSO-ETM8 : Subsystem
  PSO-ETM9 : Subsystem
  Radial Basis Network1 : Subsystem
      mask help: Radial Basis Network
      mask Display: e = 0.06;c1 = [120 150 230]/255;c2 = ([120 150 230]+0)/383;c3 = ([120 150 230]+128)/383;patch([0 1 1 0],[0 0 1 1],c1);patch([0 1 1 1-e 1-e 0+e],[0 0 1 1-e 0+e 0+e],c2);patch([0 0 1 1-e 0+e 0+e],[0 1 1 1-e 1-e 0+e],c3);plot([0 1 1 0 0],[0 0 1 1 0]);fprintf('NNET');port_label('input',1,' Input');port_label('output',1,'Output ');
  Radians to Degrees3 : simulink_extras/Transformations/Radians to Degrees
  Radians to Degrees4 : simulink_extras/Transformations/Radians to Degrees
  Scope{1..20,23,40..48,50..53,59..70} (46 alike) : Scope
  Step{1,5,7,12,14,18,20} (7 alike) : Step  Time=0  After=x_ref  SampleTime=0
  Step3 : Step  Time=0  After=10  SampleTime=0
  Subsystem1 : Subsystem
  Subsystem2 : Subsystem
  Subsystem3 : Subsystem
  Subsystem4 : Subsystem
  Subsystem5 : Subsystem
  Subsystem6 : Subsystem
  Teta1 : Scope
  Teta2 : Scope
  To Workspace10 : ToWorkspace  VariableName=teta2_ET4  SaveFormat=Timeseries  SampleTime=-1
  To Workspace11 : ToWorkspace  VariableName=vi_tri_ET4  SaveFormat=Timeseries  SampleTime=-1
  To Workspace12 : ToWorkspace  VariableName=u_dk_ET4  SaveFormat=Timeseries  SampleTime=-1
  To Workspace13 : ToWorkspace  VariableName=teta1  SaveFormat=Timeseries  SampleTime=-1
  To Workspace14 : ToWorkspace  VariableName=teta2  SaveFormat=Timeseries  SampleTime=-1
  To Workspace15 : ToWorkspace  VariableName=Vi_tri  SaveFormat=Timeseries  SampleTime=-1
  To Workspace16 : ToWorkspace  VariableName=U_dk  SaveFormat=Timeseries  SampleTime=-1
  To Workspace4 : ToWorkspace  VariableName=Gioi_han  SaveFormat=Timeseries  SampleTime=-1
  To Workspace9 : ToWorkspace  VariableName=teta1_ET4  SaveFormat=Timeseries  SampleTime=-1
  U : Scope
  X : Scope
  ko FL2 : Subsystem
      mask help: Radial Basis Network
      mask Display: e = 0.06;c1 = [120 150 230]/255;c2 = ([120 150 230]+0)/383;c3 = ([120 150 230]+128)/383;patch([0 1 1 0],[0 0 1 1],c1);patch([0 1 1 1-e 1-e 0+e],[0 0 1 1-e 0+e 0+e],c2);patch([0 0 1 1-e 0+e 0+e],[0 1 1 1-e 1-e 0+e],c3);plot([0 1 1 0 0],[0 0 1 1 0]);fprintf('NNET');port_label('input',1,' Input');port_label('output',1,'Output ');
  ko co FL_26.1_1 : Subsystem
      mask help: Radial Basis Network
      mask Display: e = 0.06;c1 = [120 150 230]/255;c2 = ([120 150 230]+0)/383;c3 = ([120 150 230]+128)/383;patch([0 1 1 0],[0 0 1 1],c1);patch([0 1 1 1-e 1-e 0+e],[0 0 1 1-e 0+e 0+e],c2);patch([0 0 1 1-e 0+e 0+e],[0 1 1 1-e 1-e 0+e],c3);plot([0 1 1 0 0],[0 0 1 1 0]);fprintf('NNET');port_label('input',1,' Input');port_label('output',1,'Output ');
  wires:
  ADRC 2/1(u) -> "Ko co bx, bl, bc-2"/2(Fl), Scope17/1  "ADRC"
  ADRC 11/1(u) -> "Ko co bx, bl, bc-1"/2(Fl), Scope19/1  "ADRC"
  ADRC 1/1(u) -> "Ko co bx, bl, bc-2"/1(Fx), To Workspace12/1, [U_dk_ET4], Scope16/1  "ADRC"
  "Ko co bx, bl, bc-2"/1(x) -> ADRC 1/2(x), To Workspace11/1, [Vi_tri_ET4], Scope8/1  "ETM4"
  "Ko co bx, bl, bc-1"/3(the1) -> Radians to Degrees3/1
  "Ko co bx, bl, bc-2"/2(l) -> [L_ET4], ADRC 2/2(x), Scope9/1  "Length"
  "Ko co bx, bl, bc-1"/1(x) -> ADRC 10/2(x), To Workspace15/1, [Vi_tri], Scope14/1  "Position"
  L_ref4/1(out) -> ADRC 11/1(ref)  "ref_ZV"
  L_ref8/1(out) -> [L_ref], ADRC 2/1(ref)  "ref_ZV"
  "Ko co bx, bl, bc-1"/2(l) -> Scope15/1, ADRC 11/2(x), [L_nIS]  "Length"
  Step7/1 -> ADRC 10/1(ref)  "ref_ZV"
  Gain4/1 -> To Workspace9/1, [Teta1_ET4], Scope10/1
  ETM2/1(ref_ETM4) -> ADRC 1/1(ref), Scope23/1  "ref_ZV"
  Step5/1 -> [x_ref], ETM2/1(ref_ETm4)  "ref_ZV"
  ADRC 10/1(u) -> "Ko co bx, bl, bc-1"/1(Fx), To Workspace16/1, [U_dk], Scope18/1  "ADRC"
  Radians to Degrees3/1 -> To Workspace13/1, [Teta1], Scope12/1
  "Ko co bx, bl, bc-1"/4(the2) -> Radians to Degrees4/1
  "Ko co bx, bl, bc-2"/3(the1) -> Gain4/1
  Gain1/1 -> To Workspace10/1, [Teta2_ET4], Scope11/1
  "Ko co bx, bl, bc-2"/4(the2) -> Gain1/1
  Radians to Degrees4/1 -> [Teta2], To Workspace14/1, Scope13/1
  [Teta2] -> Mux1/1  "nIS"
  [U_dk] -> Mux3/1  "nIS"
  [U_dk_ET4] -> Mux3/2  "ET4"
  [Teta2_ET4] -> Mux1/2  "ET4_non NN"
  [Teta1] -> Mux/1  "nIS"
  Mux2/1 -> X/1
  Mux/1 -> Teta1/1
  Mux1/1 -> Teta2/1
  Mux3/1 -> U/1
  [Teta1_ET4] -> Mux/2  "ET4_non NN"
  Step3/1 -> To Workspace4/1
  Mux7/1 -> L/1
  "Ko co bx, bl, bc-3"/3(the1) -> Gain11/1
  "Ko co bx, bl, bc-3"/1(x) -> ADRC 9/2(x), [Vi_tri_ET4_LT2bo], Scope46/1  "PSO"
  ADRC 9/1(u) -> "Ko co bx, bl, bc-3"/1(Fx), [U_dk_ET4_LT2bo], Scope44/1  "ADRC"
  Gain12/1 -> [Teta2_ET4_LT2bo], Scope41/1
  ADRC 12/1(u) -> "Ko co bx, bl, bc-3"/2(Fl), Scope45/1  "ADRC"
  Demux4/3 -> PSO-ETM5/4(Input2)
  PSO-ETM6/1(ref) -> ADRC 9/1(ref), Scope43/1  "ref_ZV"
  "Ko co bx, bl, bc-3"/4(the2) -> Gain12/1
  Step12/1 -> PSO-ETM5/1(In1)  "ref_ZV"
  Demux5/2 -> PSO-ETM6/3(Input1)
  Demux4/2 -> PSO-ETM5/3(Input1)
  Constant3/1 -> Mux8/2
  Gain11/1 -> [Teta1_ET4_LT2bo], Scope40/1
  Demux5/3 -> PSO-ETM6/4(Input2)
  "Ko co bx, bl, bc-3"/2(l) -> Scope47/1, [L_ET4_LT2bo], ADRC 12/2(x), Mux8/1  "Length"
  PSO-ETM5/1(Out1) -> PSO-ETM6/1(In1), Scope42/1  "ref_ZV"
  Demux4/1 -> PSO-ETM5/2(Input)
  Mux8/1 -> Bo2_LT_1/1(Input), Bo1_LT_1/1(Input)
  Demux5/1 -> PSO-ETM6/2(Input)
  L_ref1/1(out) -> ADRC 12/1(ref)  "ref_ZV"
  Demux2/1 -> Display3/1, PSO-ETM2/2(Input)
  ADRC 13/1(u) -> "Ko co bx, bl, bc-4"/2(Fl), Scope51/1  "ADRC"
  Constant4/1 -> Mux9/2
  "Ko co bx, bl, bc-4"/2(l) -> Scope53/1, [L_ET4_LTbo1], ADRC 13/2(x), Mux9/1  "Length"
  Demux2/2 -> Display1/1, PSO-ETM2/3(Input1)
  L_ref2/1(out) -> ADRC 13/1(ref)  "ref_ZV"
  Step14/1 -> PSO-ETM2/1(In1)  "ref_ZV"
  Mux9/1 -> Bo1_LT_2/1(Input)
  Demux2/3 -> Display2/1, PSO-ETM2/4(Input2)
  "Ko co bx, bl, bc-4"/4(the2) -> Gain6/1
  PSO-ETM2/1(ref) -> ADRC 14/1(ref), Scope48/1  "ref_"
  Gain5/1 -> [Teta1_ET4_LTbo1], Scope7/1
  Gain6/1 -> [Teta2_ET4_LTbo1], Scope20/1
  "Ko co bx, bl, bc-4"/3(the1) -> Gain5/1
  ADRC 14/1(u) -> Scope50/1, "Ko co bx, bl, bc-4"/1(Fx), [U_dk_ET4_LTbo1]  "ADRC"
  "Ko co bx, bl, bc-4"/1(x) -> ADRC 14/2(x), [Vi_tri_ET4_LTbo1], Scope52/1  "PSO"
  Bo1_LT_2/1(Output) -> Demux2/1
  Demux7/3 -> PSO-ETM8/4(Input2)
  Demux7/1 -> PSO-ETM8/2(Input)
  Gain16/1 -> [Teta2_PSO_bo1], Scope60/1
  "Ko co bx, bl, bc-5"/4(the2) -> Gain16/1
  "Ko co bx, bl, bc-5"/3(the1) -> Gain15/1
  Constant6/1 -> Mux11/2
  Gain15/1 -> [Teta1_PSO_bo1], Scope59/1
  Demux7/2 -> PSO-ETM8/3(Input1)
  "Ko co bx, bl, bc-5"/2(l) -> Scope64/1, [L_PSO_bo1], ADRC 18/2(x), Mux11/1  "Length"
  L_ref3/1(out) -> ADRC 18/1(ref)  "ref_ZV"
  PSO-ETM8/1(ref) -> ADRC 17/1(ref)  "ref_ZV"
  Step18/1 -> PSO-ETM8/1(In1)  "ref_ZV"
  ADRC 17/1(u) -> Scope61/1, "Ko co bx, bl, bc-5"/1(Fx), [U_dk_PSO_bo1]  "ADRC"
  "Ko co bx, bl, bc-5"/1(x) -> ADRC 17/2(x), [Vi_tri_PSO_bo1], Scope63/1  "PSO"
  ADRC 18/1(u) -> "Ko co bx, bl, bc-5"/2(Fl), Scope62/1  "ADRC"
  "Ko co bx, bl, bc-6"/1(x) -> ADRC 19/2(x), [Vi_tri_PSO_2bo], Scope69/1  "PSO"
  ADRC 19/1(u) -> Scope67/1, "Ko co bx, bl, bc-6"/1(Fx), [U_dk_PSO_2bo]  "ADRC"
  "Ko co bx, bl, bc-6"/2(l) -> Scope70/1, [L_PSO_2bo], ADRC 20/2(x), Mux12/1  "Length"
  L_ref5/1(out) -> ADRC 20/1(ref)  "ref_ZV"
  Step20/1 -> PSO-ETM9/1(In1)  "ref_ZV"
  "Ko co bx, bl, bc-6"/4(the2) -> Gain18/1
  "Ko co bx, bl, bc-6"/3(the1) -> Gain17/1
  Gain17/1 -> [Teta1_PSO_2bo], Scope65/1
  Gain18/1 -> [Teta2_PSO_2bo], Scope66/1
  Constant7/1 -> Mux12/2
  ADRC 20/1(u) -> "Ko co bx, bl, bc-6"/2(Fl), Scope68/1  "ADRC"
  Bo1_LT_1/1(Output) -> Display9/1, Demux4/1
  Radial Basis Network1/1(Output) -> Display/1, Demux7/1
  Mux11/1 -> Radial Basis Network1/1(Input)
  Demux8/1 -> PSO-ETM9/2(Input)
  Demux8/2 -> PSO-ETM9/3(Input1)
  Demux8/3 -> PSO-ETM9/4(Input2)
  [Teta1_ET4_LTbo1] -> Subsystem5/1(e)
  Subsystem4/1(Out1) -> Display19/1  "PSO 2 bo_non FL"
  [Teta2_ET4_LT2bo] -> Subsystem1/2(e1)
  [Teta2_PSO_bo1] -> Subsystem3/2(e1)
  Subsystem5/1(Out1) -> Display20/1  "LT chi bo 1"
  [Teta2_ET4_LTbo1] -> Subsystem5/2(e1)
  [Teta1_PSO_2bo] -> Subsystem4/1(e)
  [Teta2_PSO_2bo] -> Subsystem4/2(e1)
  Subsystem1/1(Out1) -> Display12/1  "Data_LT_2 bo"
  Subsystem3/1(Out1) -> Display18/1  "PSO chi bo 1"
  [Teta1_PSO_bo1] -> Subsystem3/1(e)
  [Teta1_ET4_LT2bo] -> Subsystem1/1(e)
  Bo2_LT_2/1(Output) -> Demux9/1
  Demux9/2 -> PSO-ETM7/3(Input1)
  Mux12/1 -> ko co FL_26.1_1/1(Input), Bo2_LT_2/1(Input)
  Demux9/3 -> PSO-ETM7/4(Input2)
  Demux9/1 -> PSO-ETM7/2(Input)
  PSO-ETM9/1(ref) -> PSO-ETM7/1(In1)  "ref_"
  PSO-ETM7/1(ref) -> ADRC 19/1(ref)  "ref_ZV"
  [Teta1_ET4_LT2bo] -> Mux/3  "Data_LT_2bo"
  [Teta1_ET4_LTbo1] -> Mux/4  "Data_LT_bo 1"
  [Teta1_PSO_2bo] -> Mux/5  "PSO_2bo"
  [Teta1_PSO_bo1] -> Mux/6  "PSO_bo1"
  [Teta2_ET4_LT2bo] -> Mux1/3  "Data_LT_2bo"
  [Teta2_ET4_LTbo1] -> Mux1/4  "Data_LT_bo 1"
  [Teta2_PSO_2bo] -> Mux1/5  "PSO_2bo"
  [Teta2_PSO_bo1] -> Mux1/6  "PSO_bo1"
  [x_ref] -> Mux2/1  "REF"
  [Vi_tri] -> Mux2/2  "nIS"
  [Vi_tri_ET4] -> Mux2/3  "ET4_non ANN"
  [Vi_tri_ET4_LT2bo] -> Mux2/4  "Data_LT_2bo"
  [Vi_tri_ET4_LTbo1] -> Mux2/5  "Data_LT_bo 1"
  [Vi_tri_PSO_2bo] -> Mux2/6  "PSO_2bo"
  [Vi_tri_PSO_bo1] -> Mux2/7  "PSO_bo1"
  [U_dk_ET4_LT2bo] -> Mux3/3  "Data_LT_2bo"
  [U_dk_ET4_LTbo1] -> Mux3/4  "Data_LT_bo 1"
  [U_dk_PSO_2bo] -> Mux3/5  "PSO_2bo"
  [U_dk_PSO_bo1] -> Mux3/6  "PSO_bo1"
  [L_ref] -> Mux7/1  "REF"
  [L_nIS] -> Mux7/2  "nIS"
  [L_ET4] -> Mux7/3  "ET4"
  [L_ET4_LT2bo] -> Mux7/4  "Data_LT_2bo"
  [L_ET4_LTbo1] -> Mux7/5  "Data_LT_bo 1"
  [L_PSO_2bo] -> Mux7/6  "PSO_2bo"
  [L_PSO_bo1] -> Mux7/7  "PSO_bo1"
  [Teta1_ET4] -> Subsystem2/1(e)
  [Teta2_ET4] -> Subsystem2/2(e1)
  Subsystem2/1(Out1) -> Display4/1  "ET4"
  ko co FL_26.1_1/1(Output) -> Display6/1, Demux8/1
  "Ko co bx, bl, bc-7"/4(the2) -> Gain3/1
  Demux1/2 -> PSO-ETM3/3(Input1)
  PSO-ETM3/1(ref) -> PSO-ETM1/1(In1)  "ref_"
  ADRC 4/1(u) -> "Ko co bx, bl, bc-7"/2(Fl), Scope4/1  "ADRC"
  Constant1/1 -> Mux4/2
  Co FL/1(Output) -> Display7/1, Demux1/1
  Demux1/1 -> PSO-ETM3/2(Input)
  Demux1/3 -> PSO-ETM3/4(Input2)
  Gain3/1 -> [Teta2_PSO_2bo_FL], Scope2/1
  L_ref6/1(out) -> ADRC 4/1(ref)  "ref_ZV"
  Gain2/1 -> [Teta1_PSO_2bo_FL], Scope1/1
  "Ko co bx, bl, bc-7"/2(l) -> Scope6/1, [L_PSO_2bo_FL], ADRC 4/2(x), Mux4/1  "Length"
  "Ko co bx, bl, bc-7"/3(the1) -> Gain2/1
  "Ko co bx, bl, bc-7"/1(x) -> ADRC 3/2(x), [Vi_tri_PSO_2bo_FL], Scope5/1  "PSO"
  Step1/1 -> PSO-ETM3/1(In1)  "ref_ZV"
  Demux3/1 -> PSO-ETM1/2(Input)
  PSO-ETM1/1(ref) -> ADRC 3/1(ref)  "ref_ZV"
  ADRC 3/1(u) -> Scope3/1, "Ko co bx, bl, bc-7"/1(Fx), [U_dk_PSO_2bo_FL]  "ADRC"
  Demux3/3 -> PSO-ETM1/4(Input2)
  Mux4/1 -> Bo2_LT_3/1(Input), Co FL/1(Input)
  Demux3/2 -> PSO-ETM1/3(Input1)
  Bo2_LT_3/1(Output) -> Demux3/1
  [Teta2_PSO_2bo_FL] -> Subsystem6/2(e1)
  Subsystem6/1(Out1) -> Display5/1  "PSO 2 bo_FL"
  [Teta1_PSO_2bo_FL] -> Subsystem6/1(e)
  [Teta1_PSO_2bo_FL] -> Mux/7
  [Teta2_PSO_2bo_FL] -> Mux1/7
  Bo2_LT_1/1(Output) -> Display8/1, Demux5/1

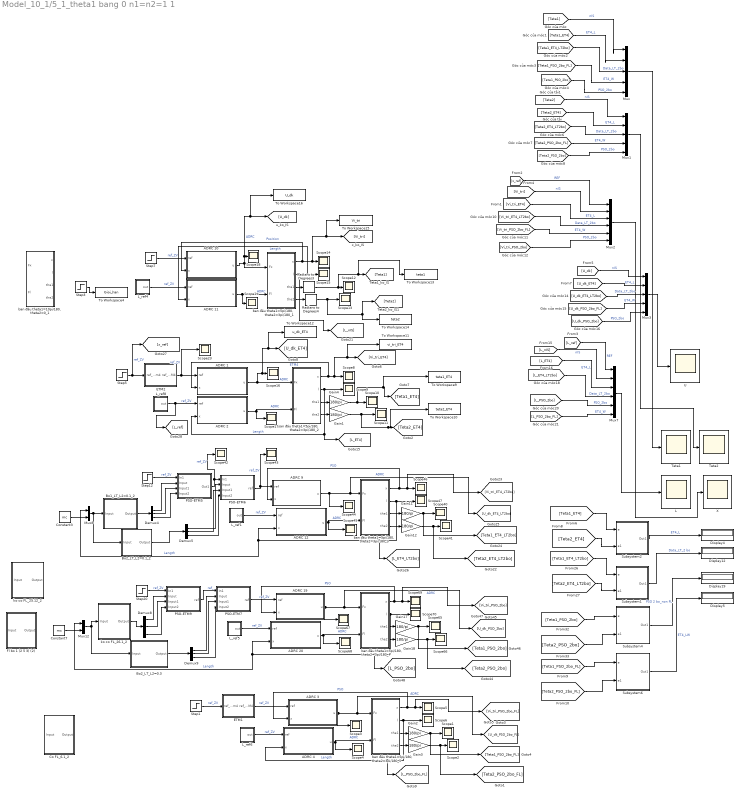
== system Model_10_1/5_1_theta1 bang 0 n1=n2=1 1 ==
  " ban đầu theta1=10pi/180, theta2=0_1" : Subsystem
  ADRC 1 : Subsystem
  ADRC 10 : Subsystem
  ADRC 11 : Subsystem
  ADRC 12 : Subsystem
  ADRC 19 : Subsystem
  ADRC 2 : Subsystem
  ADRC 20 : Subsystem
  ADRC 3 : Subsystem
  ADRC 4 : Subsystem
  ADRC 9 : Subsystem
  Bo1_LT_L2=0.1_2 : Subsystem
      mask help: Radial Basis Network
      mask Display: e = 0.06;c1 = [120 150 230]/255;c2 = ([120 150 230]+0)/383;c3 = ([120 150 230]+128)/383;patch([0 1 1 0],[0 0 1 1],c1);patch([0 1 1 1-e 1-e 0+e],[0 0 1 1-e 0+e 0+e],c2);patch([0 0 1 1-e 0+e 0+e],[0 1 1 1-e 1-e 0+e],c3);plot([0 1 1 0 0],[0 0 1 1 0]);fprintf('NNET');port_label('input',1,' Input');port_label('output',1,'Output ');
  Bo2_LT_L2=0.1_2 : Subsystem
      mask help: Radial Basis Network
      mask Display: e = 0.06;c1 = [120 150 230]/255;c2 = ([120 150 230]+0)/383;c3 = ([120 150 230]+128)/383;patch([0 1 1 0],[0 0 1 1],c1);patch([0 1 1 1-e 1-e 0+e],[0 0 1 1-e 0+e 0+e],c2);patch([0 0 1 1-e 0+e 0+e],[0 1 1 1-e 1-e 0+e],c3);plot([0 1 1 0 0],[0 0 1 1 0]);fprintf('NNET');port_label('input',1,' Input');port_label('output',1,'Output ');
  Bo2_LT_L2=0.3 : Subsystem
      mask help: Radial Basis Network
      mask Display: e = 0.06;c1 = [120 150 230]/255;c2 = ([120 150 230]+0)/383;c3 = ([120 150 230]+128)/383;patch([0 1 1 0],[0 0 1 1],c1);patch([0 1 1 1-e 1-e 0+e],[0 0 1 1-e 0+e 0+e],c2);patch([0 0 1 1-e 0+e 0+e],[0 1 1 1-e 1-e 0+e],c3);plot([0 1 1 0 0],[0 0 1 1 0]);fprintf('NNET');port_label('input',1,' Input');port_label('output',1,'Output ');
  Co FL_6.1_2 : Subsystem
      mask help: Radial Basis Network
      mask Display: e = 0.06;c1 = [120 150 230]/255;c2 = ([120 150 230]+0)/383;c3 = ([120 150 230]+128)/383;patch([0 1 1 0],[0 0 1 1],c1);patch([0 1 1 1-e 1-e 0+e],[0 0 1 1-e 0+e 0+e],c2);patch([0 0 1 1-e 0+e 0+e],[0 1 1 1-e 1-e 0+e],c3);plot([0 1 1 0 0],[0 0 1 1 0]);fprintf('NNET');port_label('input',1,' Input');port_label('output',1,'Output ');
  Constant3 : Constant  Value=mc
  Constant7 : Constant  Value=mc
  Demux{4..5,8..9} (4 alike) : Demux  Outputs=3
  Display{4..5,12,19} (4 alike) : Display
  ETM1 : Subsystem
  ETM2 : Subsystem
  Fl bo 1 (2 5 3) (2) : Subsystem
      mask help: Radial Basis Network
      mask Display: e = 0.06;c1 = [120 150 230]/255;c2 = ([120 150 230]+0)/383;c3 = ([120 150 230]+128)/383;patch([0 1 1 0],[0 0 1 1],c1);patch([0 1 1 1-e 1-e 0+e],[0 0 1 1-e 0+e 0+e],c2);patch([0 0 1 1-e 0+e 0+e],[0 1 1 1-e 1-e 0+e],c3);plot([0 1 1 0 0],[0 0 1 1 0]);fprintf('NNET');port_label('input',1,' Input');port_label('output',1,'Output ');
  Gain{1..4,11..12,17..18} (8 alike) : Gain  Gain=180/pi
  L : Scope
  L_ref1 : Subsystem
  L_ref4 : Subsystem
  L_ref5 : Subsystem
  L_ref6 : Subsystem
  L_ref8 : Subsystem
  Mux : Mux  Inputs=5
  Mux1 : Mux  Inputs=5
  Mux12 : Mux  Inputs=2
  Mux2 : Mux  Inputs=6
  Mux3 : Mux  Inputs=5
  Mux7 : Mux  Inputs=6
  Mux8 : Mux  Inputs=2
  PSO-ETM5 : Subsystem
  PSO-ETM6 : Subsystem
  PSO-ETM7 : Subsystem
  PSO-ETM9 : Subsystem
  Radians to Degrees3 : simulink_extras/Transformations/Radians to Degrees
  Radians to Degrees4 : simulink_extras/Transformations/Radians to Degrees
  Scope{1..6,8..19,23,40..47,65..70} (33 alike) : Scope
  Step{1,5,7,12,20} (5 alike) : Step  Time=0  After=x_ref  SampleTime=0
  Step3 : Step  Time=0  After=10  SampleTime=0
  Subsystem1 : Subsystem
  Subsystem2 : Subsystem
  Subsystem4 : Subsystem
  Subsystem6 : Subsystem
  Teta1 : Scope
  Teta2 : Scope
  To Workspace10 : ToWorkspace  VariableName=teta2_ET4  SaveFormat=Timeseries  SampleTime=-1
  To Workspace11 : ToWorkspace  VariableName=vi_tri_ET4  SaveFormat=Timeseries  SampleTime=-1
  To Workspace12 : ToWorkspace  VariableName=u_dk_ET4  SaveFormat=Timeseries  SampleTime=-1
  To Workspace13 : ToWorkspace  VariableName=teta1  SaveFormat=Timeseries  SampleTime=-1
  To Workspace14 : ToWorkspace  VariableName=teta2  SaveFormat=Timeseries  SampleTime=-1
  To Workspace15 : ToWorkspace  VariableName=Vi_tri  SaveFormat=Timeseries  SampleTime=-1
  To Workspace16 : ToWorkspace  VariableName=U_dk  SaveFormat=Timeseries  SampleTime=-1
  To Workspace4 : ToWorkspace  VariableName=Gioi_han  SaveFormat=Timeseries  SampleTime=-1
  To Workspace9 : ToWorkspace  VariableName=teta1_ET4  SaveFormat=Timeseries  SampleTime=-1
  U : Scope
  X : Scope
  "ban đầu theta1=5pi/180, theta2=3pi/180_1" : Subsystem
  "ban đầu theta1=5pi/180, theta2=3pi/180_2" : Subsystem
  "ban đầu theta1=5pi/180, theta2=3pi/180_3" : Subsystem
  "ban đầu theta1=5pi/180, theta2=3pi/180_4" : Subsystem
  "ban đầu theta1=5pi/180, theta2=3pi/180_5" : Subsystem
  ko co FL_25.12_2 : Subsystem
      mask help: Radial Basis Network
      mask Display: e = 0.06;c1 = [120 150 230]/255;c2 = ([120 150 230]+0)/383;c3 = ([120 150 230]+128)/383;patch([0 1 1 0],[0 0 1 1],c1);patch([0 1 1 1-e 1-e 0+e],[0 0 1 1-e 0+e 0+e],c2);patch([0 0 1 1-e 0+e 0+e],[0 1 1 1-e 1-e 0+e],c3);plot([0 1 1 0 0],[0 0 1 1 0]);fprintf('NNET');port_label('input',1,' Input');port_label('output',1,'Output ');
  ko co FL_26.1_2 : Subsystem
      mask help: Radial Basis Network
      mask Display: e = 0.06;c1 = [120 150 230]/255;c2 = ([120 150 230]+0)/383;c3 = ([120 150 230]+128)/383;patch([0 1 1 0],[0 0 1 1],c1);patch([0 1 1 1-e 1-e 0+e],[0 0 1 1-e 0+e 0+e],c2);patch([0 0 1 1-e 0+e 0+e],[0 1 1 1-e 1-e 0+e],c3);plot([0 1 1 0 0],[0 0 1 1 0]);fprintf('NNET');port_label('input',1,' Input');port_label('output',1,'Output ');
  wires:
  ADRC 2/1(u) -> "ban đầu theta1=5pi/180, theta2=3pi/180_2"/2(Fl), Scope17/1  "ADRC"
  ADRC 11/1(u) -> "ban đầu theta1=5pi/180, theta2=3pi/180_1"/2(Fl), Scope19/1  "ADRC"
  ADRC 1/1(u) -> "ban đầu theta1=5pi/180, theta2=3pi/180_2"/1(Fx), To Workspace12/1, [U_dk_ET4], Scope16/1  "ADRC"
  "ban đầu theta1=5pi/180, theta2=3pi/180_2"/1(x) -> ADRC 1/2(x), To Workspace11/1, [Vi_tri_ET4], Scope8/1  "ETM4"
  "ban đầu theta1=5pi/180, theta2=3pi/180_1"/3(the1) -> Radians to Degrees3/1
  "ban đầu theta1=5pi/180, theta2=3pi/180_2"/2(l) -> [L_ET4], ADRC 2/2(x), Scope9/1  "Length"
  "ban đầu theta1=5pi/180, theta2=3pi/180_1"/1(x) -> ADRC 10/2(x), To Workspace15/1, [Vi_tri], Scope14/1  "Position"
  L_ref4/1(out) -> ADRC 11/1(ref)  "ref_ZV"
  L_ref8/1(out) -> [L_ref], ADRC 2/1(ref)  "ref_ZV"
  "ban đầu theta1=5pi/180, theta2=3pi/180_1"/2(l) -> Scope15/1, ADRC 11/2(x), [L_nIS]  "Length"
  Step7/1 -> ADRC 10/1(ref)  "ref_ZV"
  Gain4/1 -> To Workspace9/1, [Teta1_ET4], Scope10/1
  ETM2/1(ref_ETM4) -> ADRC 1/1(ref), Scope23/1  "ref_ZV"
  Step5/1 -> [x_ref], ETM2/1(ref_ETm4)  "ref_ZV"
  ADRC 10/1(u) -> "ban đầu theta1=5pi/180, theta2=3pi/180_1"/1(Fx), To Workspace16/1, [U_dk], Scope18/1  "ADRC"
  Radians to Degrees3/1 -> To Workspace13/1, [Teta1], Scope12/1
  "ban đầu theta1=5pi/180, theta2=3pi/180_1"/4(the2) -> Radians to Degrees4/1
  "ban đầu theta1=5pi/180, theta2=3pi/180_2"/3(the1) -> Gain4/1
  Gain1/1 -> To Workspace10/1, [Teta2_ET4], Scope11/1
  "ban đầu theta1=5pi/180, theta2=3pi/180_2"/4(the2) -> Gain1/1
  Radians to Degrees4/1 -> [Teta2], To Workspace14/1, Scope13/1
  [Teta2] -> Mux1/1  "nIS"
  [U_dk] -> Mux3/1  "nIS"
  [U_dk_ET4] -> Mux3/2  "ET4_L"
  [Teta2_ET4] -> Mux1/2  "ET4_L"
  [Teta1] -> Mux/1  "nIS"
  Mux2/1 -> X/1
  Mux/1 -> Teta1/1
  Mux1/1 -> Teta2/1
  Mux3/1 -> U/1
  [Teta1_ET4] -> Mux/2  "ET4_L"
  Step3/1 -> To Workspace4/1
  Mux7/1 -> L/1
  "ban đầu theta1=5pi/180, theta2=3pi/180_3"/3(the1) -> Gain11/1
  "ban đầu theta1=5pi/180, theta2=3pi/180_3"/1(x) -> ADRC 9/2(x), [Vi_tri_ET4_LT2bo], Scope46/1  "PSO"
  ADRC 9/1(u) -> "ban đầu theta1=5pi/180, theta2=3pi/180_3"/1(Fx), [U_dk_ET4_LT2bo], Scope44/1  "ADRC"
  Gain12/1 -> [Teta2_ET4_LT2bo], Scope41/1
  ADRC 12/1(u) -> "ban đầu theta1=5pi/180, theta2=3pi/180_3"/2(Fl), Scope45/1  "ADRC"
  Demux4/3 -> PSO-ETM5/4(Input2)
  PSO-ETM6/1(ref) -> ADRC 9/1(ref), Scope43/1  "ref_ZV"
  "ban đầu theta1=5pi/180, theta2=3pi/180_3"/4(the2) -> Gain12/1
  Step12/1 -> PSO-ETM5/1(In1)  "ref_ZV"
  Demux5/2 -> PSO-ETM6/3(Input1)
  Demux4/2 -> PSO-ETM5/3(Input1)
  Constant3/1 -> Mux8/2
  Gain11/1 -> [Teta1_ET4_LT2bo], Scope40/1
  Demux5/3 -> PSO-ETM6/4(Input2)
  "ban đầu theta1=5pi/180, theta2=3pi/180_3"/2(l) -> Scope47/1, [L_ET4_LT2bo], ADRC 12/2(x), Mux8/1  "Length"
  Bo2_LT_L2=0.1_2/1(Output) -> Demux5/1
  PSO-ETM5/1(Out1) -> PSO-ETM6/1(In1), Scope42/1  "ref_ZV"
  Demux4/1 -> PSO-ETM5/2(Input)
  Mux8/1 -> Bo2_LT_L2=0.1_2/1(Input), Bo1_LT_L2=0.1_2/1(Input)
  Demux5/1 -> PSO-ETM6/2(Input)
  L_ref1/1(out) -> ADRC 12/1(ref)  "ref_ZV"
  "ban đầu theta1=5pi/180, theta2=3pi/180_4"/1(x) -> ADRC 19/2(x), [Vi_tri_PSO_2bo], Scope69/1  "PSO"
  ADRC 19/1(u) -> Scope67/1, "ban đầu theta1=5pi/180, theta2=3pi/180_4"/1(Fx), [U_dk_PSO_2bo]  "ADRC"
  "ban đầu theta1=5pi/180, theta2=3pi/180_4"/2(l) -> Scope70/1, [L_PSO_2bo], ADRC 20/2(x), Mux12/1  "Length"
  L_ref5/1(out) -> ADRC 20/1(ref)  "ref_ZV"
  Step20/1 -> PSO-ETM9/1(In1)  "ref_ZV"
  "ban đầu theta1=5pi/180, theta2=3pi/180_4"/4(the2) -> Gain18/1
  "ban đầu theta1=5pi/180, theta2=3pi/180_4"/3(the1) -> Gain17/1
  Gain17/1 -> [Teta1_PSO_2bo], Scope65/1
  Gain18/1 -> [Teta2_PSO_2bo], Scope66/1
  Constant7/1 -> Mux12/2
  ADRC 20/1(u) -> "ban đầu theta1=5pi/180, theta2=3pi/180_4"/2(Fl), Scope68/1  "ADRC"
  Bo1_LT_L2=0.1_2/1(Output) -> Demux4/1
  Demux8/1 -> PSO-ETM9/2(Input)
  Demux8/2 -> PSO-ETM9/3(Input1)
  Demux8/3 -> PSO-ETM9/4(Input2)
  Subsystem4/1(Out1) -> Display19/1  "PSO 2 bo_non FL"
  [Teta2_ET4_LT2bo] -> Subsystem1/2(e1)
  [Teta1_PSO_2bo] -> Subsystem4/1(e)
  [Teta2_PSO_2bo] -> Subsystem4/2(e1)
  Subsystem1/1(Out1) -> Display12/1  "Data_LT_2 bo"
  [Teta1_ET4_LT2bo] -> Subsystem1/1(e)
  Bo2_LT_L2=0.3/1(Output) -> Demux9/1
  Demux9/2 -> PSO-ETM7/3(Input1)
  Mux12/1 -> ko co FL_26.1_2/1(Input), Bo2_LT_L2=0.3/1(Input)
  Demux9/3 -> PSO-ETM7/4(Input2)
  Demux9/1 -> PSO-ETM7/2(Input)
  PSO-ETM9/1(ref) -> PSO-ETM7/1(In1)  "ref_"
  PSO-ETM7/1(ref) -> ADRC 19/1(ref)  "ref_ZV"
  [Teta1_ET4_LT2bo] -> Mux/3  "Data_LT_2bo"
  [Teta1_PSO_2bo_FL] -> Mux/4  "ET4_W"
  [Teta1_PSO_2bo] -> Mux/5  "PSO_2bo"
  [Teta2_ET4_LT2bo] -> Mux1/3  "Data_LT_2bo"
  [Teta2_PSO_2bo_FL] -> Mux1/4  "ET4_W"
  [Teta2_PSO_2bo] -> Mux1/5  "PSO_2bo"
  [x_ref] -> Mux2/1  "REF"
  [Vi_tri] -> Mux2/2  "nIS"
  [Vi_tri_ET4] -> Mux2/3  "ET4_L"
  [Vi_tri_ET4_LT2bo] -> Mux2/4  "Data_LT_2bo"
  [Vi_tri_PSO_2bo_FL] -> Mux2/5  "ET4_W"
  [Vi_tri_PSO_2bo] -> Mux2/6  "PSO_2bo"
  [U_dk_ET4_LT2bo] -> Mux3/3  "Data_LT_2bo"
  [U_dk_PSO_2bo_FL] -> Mux3/4  "ET4_W"
  [U_dk_PSO_2bo] -> Mux3/5  "PSO_2bo"
  [L_ref] -> Mux7/1  "REF"
  [L_nIS] -> Mux7/2  "nIS"
  [L_ET4] -> Mux7/3  "ET4_L"
  [L_ET4_LT2bo] -> Mux7/4  "Data_LT_2bo"
  [Teta1_ET4] -> Subsystem2/1(e)
  [Teta2_ET4] -> Subsystem2/2(e1)
  Subsystem2/1(Out1) -> Display4/1  "ET4_L"
  "ban đầu theta1=5pi/180, theta2=3pi/180_5"/4(the2) -> Gain3/1
  ADRC 4/1(u) -> "ban đầu theta1=5pi/180, theta2=3pi/180_5"/2(Fl), Scope4/1  "ADRC"
  Gain3/1 -> [Teta2_PSO_2bo_FL], Scope2/1
  L_ref6/1(out) -> ADRC 4/1(ref)  "ref_ZV"
  Gain2/1 -> [Teta1_PSO_2bo_FL], Scope1/1
  "ban đầu theta1=5pi/180, theta2=3pi/180_5"/2(l) -> Scope6/1, [L_PSO_2bo_FL], ADRC 4/2(x)  "Length"
  "ban đầu theta1=5pi/180, theta2=3pi/180_5"/3(the1) -> Gain2/1
  "ban đầu theta1=5pi/180, theta2=3pi/180_5"/1(x) -> ADRC 3/2(x), [Vi_tri_PSO_2bo_FL], Scope5/1  "PSO"
  Step1/1 -> ETM1/1(ref_ETm4)  "ref_ZV"
  ETM1/1(ref_ETM4) -> ADRC 3/1(ref)  "ref_ZV"
  ADRC 3/1(u) -> Scope3/1, "ban đầu theta1=5pi/180, theta2=3pi/180_5"/1(Fx), [U_dk_PSO_2bo_FL]  "ADRC"
  [Teta2_PSO_2bo_FL] -> Subsystem6/2(e1)
  Subsystem6/1(Out1) -> Display5/1  "ET4_LW"
  [Teta1_PSO_2bo_FL] -> Subsystem6/1(e)
  [L_PSO_2bo] -> Mux7/5  "PSO_2bo"
  [L_PSO_2bo_FL] -> Mux7/6  "ET4_W"
  ko co FL_26.1_2/1(Output) -> Demux8/1
